simulink library "CoCoSTLib"  (R2021a)
settings: Solver=ode45  StartTime=0.0  StopTime=10.0  RelTol=1e-3  EnableMultiTasking=on
values from neighbouring files (symbols this model uses):
  beta = 0.01    [var.mat]
  c = 2    [var.mat]
  m = 4    [var.mat]
  mu = 0.8    [var.mat]
  omega = 1    [var.mat]
  r = 5    [var.mat]
  s = 1.5    [var.mat]
  steadyVal = 10    [var.mat]
  zeta = 0.5    [var.mat]
undefined symbols (not defined in the file or in its folder): a, d, msgbox, T_End, T_Start, tau
libraries: $bdroot x49, simulink x4
(part 1 of 2)
settings Model: Creator=balsi  LastModifiedBy=xiayu
settings SolverCC: AlgebraicLoopSolver=TrustRegion
settings DataIOCC: LimitDataPoints=on  SaveFormat=Array  ReturnWorkspaceOutputs=off
settings OptimizationCC: LifeSpan=inf
settings DebuggingCC: SFUnexpectedBacktrackingDiag=warning  SFNoUnconditionalDefaultTransitionDiag=warning  SFExecutionAtInitializationDiag=none  SFMachineParentedDataDiag=warning  ArithmeticOperatorsInVariantConditions=warning
settings HardwareCC: ProdBitPerPointer=32  ProdBitPerSizeT=32  ProdBitPerPtrDiffT=32  ProdLargestAtomicFloat=None  ProdIntDivRoundTo=Undefined  ProdEndianess=Unspecified  ProdWordSize=32  ProdHWDeviceType=32-bit Generic
settings ModelReferenceCC: PropagateSignalLabelsOutOfModel=off
settings SFSimCC: SimUseLocalCustomCode=off  CustomCodeUndefinedFunction=UseInterfaceOnly
settings RTWCC: RTWUseLocalCustomCode=off
settings CodeAppCC: StateflowObjectComments=on
settings GRTTargetCC: TargetLangStandard=C89/C90 (ANSI)
settings ConfigComp: CovMetricSettings=dw  CovSaveCumulativeToWorkspaceVar=on  CovSaveSingleToWorkspaceVar=on  CovExternalEMLEnable=off

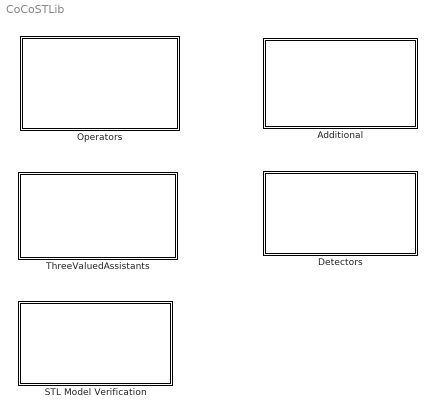
== system CoCoSTLib ==
  Additional : Subsystem
      mask Display: disp('Some Utiles')
  Detectors : Subsystem
      mask Display: disp("Detectors")
  Operators : Subsystem
      mask Display: disp("STL Operators")
  STL Model Verification : Subsystem
      mask Display: disp("STL Model Verification")
  ThreeValuedAssistants : Subsystem
      mask Display: disp("Utiles for 3V Logic")

== system CoCoSTLib/Additional ==
  note: Time Windows
  note: Latches
  note: AndSTL
  note: Delay
  AndStl_LF : Subsystem
  AndStl_LT : Subsystem
  Delay : Subsystem
  DelayedTimeWindow : Subsystem
  Latch_LF : Subsystem
  Latch_LT : Subsystem
  TimeWindow : Subsystem

== system CoCoSTLib/Detectors ==
  note: Detectors of Unaccepted signal behaviors
      |
      | - Components are in LT framework.
      | - The detectors/monitors definitions are in S T - Lib : A library for specifying and classifying model behaviors
  Overshoot : Subsystem  mask{c=c, r=r}
      mask prompts: c "Overshoot magnitude"; r "Step parameter"
      mask TypeOptions c: c/Value
      mask TypeOptions r:
      | r
      | /Value
  Ring_once : Subsystem  mask{a=a, d=2*d}
      mask prompts: a "amplitude of the ring"; d "maximum width of the ring"
      mask TypeOptions a: a/Value
      mask TypeOptions d: d/Value
  RiseTime : Subsystem  mask{r=r, zeta=zeta, value=mu * steadyVal}
      mask prompts: r "Step parameter"; zeta "Rise time"; value "Target value to reach"
      mask TypeOptions r: r/Value
      mask TypeOptions zeta: zeta/Value
      mask TypeOptions value: target value/Value
  SettlingTime : Subsystem  mask{r=r, s=s, beta=beta}
      mask prompts: r "Step parameter"; s "Settling time"; beta "Fraction of steady state value"
      mask TypeOptions r:
      | r
      | /Value
      mask TypeOptions s: s/Value
      mask TypeOptions beta: beta/Gain
  Spike : Subsystem  mask{m=m, omega=omega}
      mask prompts: m "amplitude of spike"; omega "maximum width of spike"
      mask TypeOptions m: m/Value
      mask TypeOptions omega: omega/Value
  Timed Relationship : Subsystem  mask{tau=tau}
      mask prompts: tau "Relation time"
      mask TypeOptions tau: tau/Value

== system CoCoSTLib/Operators ==
  Operators_3V : Subsystem
      mask Display: disp("Operators Three-valued Logic")
  Operators_LF : Subsystem
      mask Display: disp('Operators True Logic')
  Operators_LT : Subsystem
      mask Display: disp('Operators False Logic')

== system CoCoSTLib/STL Model Verification ==
  note: 3V assertion
  note: 3V indicator/bulb
  3V Assertion : Subsystem  mask(Assertion in Three-valued Logic){Enabled=on, AssertionFailFcn=, StopWhenAssertionFail=on}
      mask prompts: Enabled "Simulink:blkprm_prompts:AssertionEnabled"; AssertionFailFcn "Simulink:blkprm_prompts:AssertionCallback"; StopWhenAssertionFail "Simulink:blkprm_prompts:AssertionStopRequest"
      mask help:
      | The Assertion block checks whether any of the elements of the input signal are of FALSE value in Three-Valued Logic,  namely [0, 0]. If all elements are nonzero, the block does nothing. If any element is zero, the block halts the simulation, by default, and displays an error message.
      |
      | NOTE: This block is used when 3V encoding is [0, 0], [0, 1], [1, 0], [1, 1]. When 3V encoding is -1, 0, 1, use Simulink / Model Verification / Assertion.
      mask TypeOptions Enabled: Assertion/Enabled
      mask TypeOptions AssertionFailFcn: Assertion/AssertionFailFcn
      mask TypeOptions StopWhenAssertionFail: Assertion/StopWhenAssertionFail
      mask DialogControl Enabled Prompt: Enable assertion
      mask DialogControl AssertionFailFcn Prompt: Simulation callback when assertion fails:
      mask DialogControl StopWhenAssertionFail Prompt: Stop simulation when assertion fails
  3V Lamp : LampBlock
  report : Subsystem  StopFcn=msgbox('msg here', 'report');

== system CoCoSTLib/ThreeValuedAssistants ==
  note: Encoding of 3V Logic in -1, 0, 1
  note: 3V interpreter
  note: 3V assignments
  note: 3V logic operators
  AND_3V : Subsystem
  Assignment_arr : Subsystem  Commented=on
  False_3V : Subsystem
      mask Display: disp("F_3V")
  "Interpreter " : Subsystem
  NOT_3V : Subsystem
  OR_3V : Subsystem
  True_3V : Subsystem
      mask Display: disp("T_3V")
  Unknown_3V : Subsystem
      mask Display: disp("U_3V")

== system CoCoSTLib/Additional/AndStl_LF ==
  note: This block gives the time when IN has an decrease, i.e, the value of the delay
  IN : Inport
  Clock : Clock
  Constant : Constant  Value=65535  VectorParams1D=off
  Constant1 : Constant
  DetectDecrease : Subsystem
  Memory : Memory
  Memory1 : Memory
  Switch : Switch  Criteria=u2 > Threshold
  Switch1 : Switch  Criteria=u2 > Threshold
  Switch2 : Switch  Criteria=u2 > Threshold
  OUT : Outport
  wires:
  Memory1/1 -> Switch1/2, Switch2/3
  Switch/1 -> Memory/1
  Memory/1 -> Switch1/1, Switch/3
  Switch1/1 -> OUT/1
  Switch2/1 -> Memory1/1
  Clock/1 -> Switch/1
  DetectDecrease/1(Y) -> Switch/2, Switch2/2
  Constant/1 -> Switch1/3
  IN/1 -> DetectDecrease/1(U)
  Constant1/1 -> Switch2/1

== system CoCoSTLib/Additional/AndStl_LT ==
  note: This block gives the time when IN has an increase, i.e, the value of the delay
  IN : Inport
  Clock : Clock
  Constant : Constant  Value=65535
  Constant1 : Constant
  DetectIncrease : Subsystem
  Memory : Memory
  Memory1 : Memory
  Switch : Switch  Criteria=u2 > Threshold
  Switch1 : Switch  Criteria=u2 > Threshold
  Switch2 : Switch  Criteria=u2 > Threshold
  OUT : Outport
  wires:
  Clock/1 -> Switch/1
  Constant1/1 -> Switch2/1
  Memory1/1 -> Switch1/2, Switch2/3
  Switch/1 -> Memory/1
  Switch1/1 -> OUT/1
  Switch2/1 -> Memory1/1
  DetectIncrease/1(Y) -> Switch/2, Switch2/2
  IN/1 -> DetectIncrease/1(U)
  Memory/1 -> Switch1/1, Switch/3
  Constant/1 -> Switch1/3

== system CoCoSTLib/Additional/Delay ==
  T_Start : Inport
  T_End : Inport  Port=2
  Delay : Inport  Port=3
  Clock : Clock
  Compare To Constant : simulink/Logic and Bit Operations/Compare To Constant  relop=>=  const=0  OutDataTypeStr=boolean
  Constant : Constant  Value=65535
  Subtract : Sum
  Subtract1 : Sum
  Subtract2 : Sum  Inputs=-+
  Switch1 : Switch  Criteria=u2 > Threshold
  T_Start_delayed : Outport
  T_End_delayed : Outport  Port=2
  wires:
  Clock/1 -> Subtract2/2
  Constant/1 -> Switch1/3
  Switch1/1 -> Subtract/1, Subtract1/2
  Delay/1 -> Switch1/1, Subtract2/1
  T_End/1 -> Subtract1/1
  T_Start/1 -> Subtract/2
  Subtract1/1 -> T_End_delayed/1
  Subtract/1 -> T_Start_delayed/1
  Subtract2/1 -> Compare To Constant/1
  Compare To Constant/1 -> Switch1/2

== system CoCoSTLib/Additional/DelayedTimeWindow ==
  T_Start : Inport
  T_End : Inport  Port=2
  DELAY : Inport  Port=3
  AND1 : Logic  AllPortsSameDT=off  OutDataTypeStr=boolean
  CLOCK : Clock
  DELAY_SUB : Sum  Inputs=+-
  REL1 : RelationalOperator  Operator=<=  OutDataTypeStr=boolean  RndMeth=Simplest
  REL2 : RelationalOperator  Operator=<=  OutDataTypeStr=boolean  RndMeth=Simplest
  OUT : Outport
  wires:
  REL1/1 -> AND1/1
  CLOCK/1 -> DELAY_SUB/1
  REL2/1 -> AND1/2
  T_Start/1 -> REL1/1
  DELAY_SUB/1 -> REL1/2, REL2/1
  AND1/1 -> OUT/1
  DELAY/1 -> DELAY_SUB/2
  T_End/1 -> REL2/2

== system CoCoSTLib/Additional/Latch_LF ==
  In : Inport
  Memory_ini1 : Memory  InitialCondition=1
  OR : Logic  AllPortsSameDT=off  OutDataTypeStr=boolean
  Out : Outport
  wires:
  In/1 -> OR/1
  Memory_ini1/1 -> OR/2
  OR/1 -> Out/1, Memory_ini1/1

== system CoCoSTLib/Additional/Latch_LT ==
  In : Inport
  "Memory_ini0 " : Memory
  OR : Logic  Operator=OR  AllPortsSameDT=off  OutDataTypeStr=boolean
  Out : Outport
  wires:
  In/1 -> OR/1
  "Memory_ini0 "/1 -> OR/2
  OR/1 -> Out/1, "Memory_ini0 "/1

== system CoCoSTLib/Additional/TimeWindow ==
  T_Start : Inport
  T_End : Inport  Port=2
  AND : Logic  AllPortsSameDT=off  OutDataTypeStr=boolean
  CLOCK : Clock
  REL1 : RelationalOperator  Operator=<=  OutDataTypeStr=boolean  RndMeth=Simplest
  REL2 : RelationalOperator  Operator=<=  OutDataTypeStr=boolean  RndMeth=Simplest
  OUT : Outport
  wires:
  CLOCK/1 -> REL1/2, REL2/1
  T_End/1 -> REL2/2
  REL1/1 -> AND/1
  REL2/1 -> AND/2
  AND/1 -> OUT/1
  T_Start/1 -> REL1/1

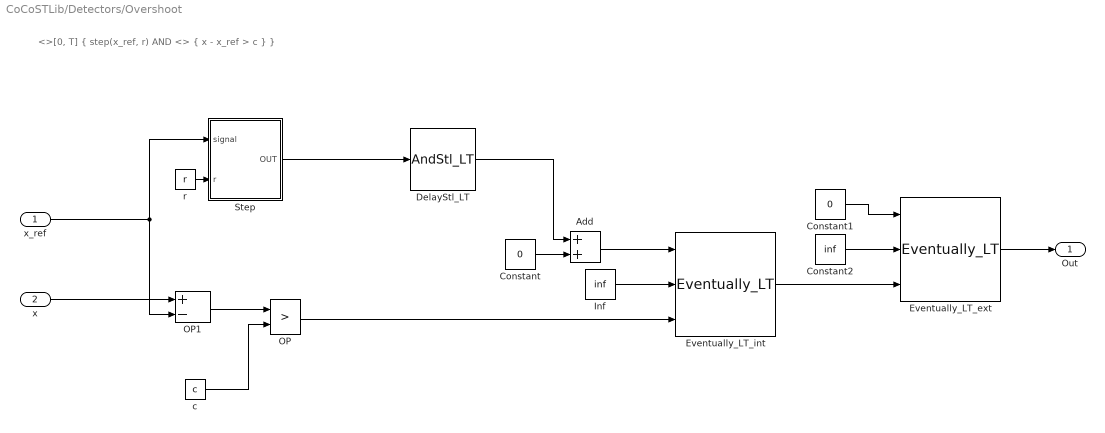
== system CoCoSTLib/Detectors/Overshoot ==
  note: <>[0, T] { step(x_ref, r) AND <> { x - x_ref > c } }
  x_ref : Inport
  x : Inport  Port=2
  Add : Sum
  Constant : Constant  Value=0
  Constant1 : Constant  Value=0
  Constant2 : Constant  Value=inf
  DelayStl_LT : $bdroot/Additional/AndStl_LT  SystemSampleTime=-1  VariantActivationTime=update diagram  Latency=0  AutoFrameSizeCalculation=off
  Eventually_LT_ext : $bdroot/Operators/Operators_LT/Eventually_LT   SystemSampleTime=-1  VariantActivationTime=update diagram  Latency=0  AutoFrameSizeCalculation=off
  "Eventually_LT_int " : $bdroot/Operators/Operators_LT/Eventually_LT   SystemSampleTime=-1  VariantActivationTime=update diagram  Latency=0  AutoFrameSizeCalculation=off
  Inf : Constant  Value=inf  OutDataTypeStr=Inherit: Inherit via back propagation
  OP : RelationalOperator  Operator=>  OutDataTypeStr=boolean  RndMeth=Simplest
  OP1 : Sum  Inputs=+-
  "Step " : Subsystem
  c : Constant  Value=c
  "r " : Constant  Value=r
  Out : Outport
  wires:
  x_ref/1 -> "Step "/1(signal), OP1/2
  DelayStl_LT/1 -> Add/1
  x/1 -> OP1/1
  Add/1 -> "Eventually_LT_int "/1
  "Step "/1(OUT) -> DelayStl_LT/1
  Eventually_LT_ext/1 -> Out/1
  "r "/1 -> "Step "/2(r)
  Constant/1 -> Add/2
  Inf/1 -> "Eventually_LT_int "/2
  c/1 -> OP/2
  Constant1/1 -> Eventually_LT_ext/1
  Constant2/1 -> Eventually_LT_ext/2
  "Eventually_LT_int "/1 -> Eventually_LT_ext/3
  OP1/1 -> OP/1
  OP/1 -> "Eventually_LT_int "/3

== system CoCoSTLib/Detectors/Ring_once ==
  note: <>[0, T] (rise and <>_[0, 2d] fall)
  signal : Inport
  "AndSTL_LT " : $bdroot/Additional/AndStl_LT  SystemSampleTime=-1  VariantActivationTime=update diagram  Latency=0  AutoFrameSizeCalculation=off
  Constant : Constant  Value=0
  "Eventually_LT " : $bdroot/Operators/Operators_LT/Eventually_LT   SystemSampleTime=-1  VariantActivationTime=update diagram  Latency=0  AutoFrameSizeCalculation=off
  Fall : Subsystem
  Rise : Subsystem
  Subtract : Sum
  Subtract1 : Sum
  a : Constant  Value=a
  d : Constant  Value=d
  "out " : Outport
  wires:
  "AndSTL_LT "/1 -> Subtract/1, Subtract1/2
  Constant/1 -> Subtract/2
  d/1 -> Subtract1/1
  Subtract/1 -> "Eventually_LT "/1
  Subtract1/1 -> "Eventually_LT "/2
  Rise/1(OUT) -> "AndSTL_LT "/1
  "Eventually_LT "/1 -> "out "/1
  signal/1 -> Fall/1(signal), Rise/1(signal)  "signal"
  Fall/1(OUT) -> "Eventually_LT "/3
  a/1 -> Rise/2("a "), Fall/2(a)

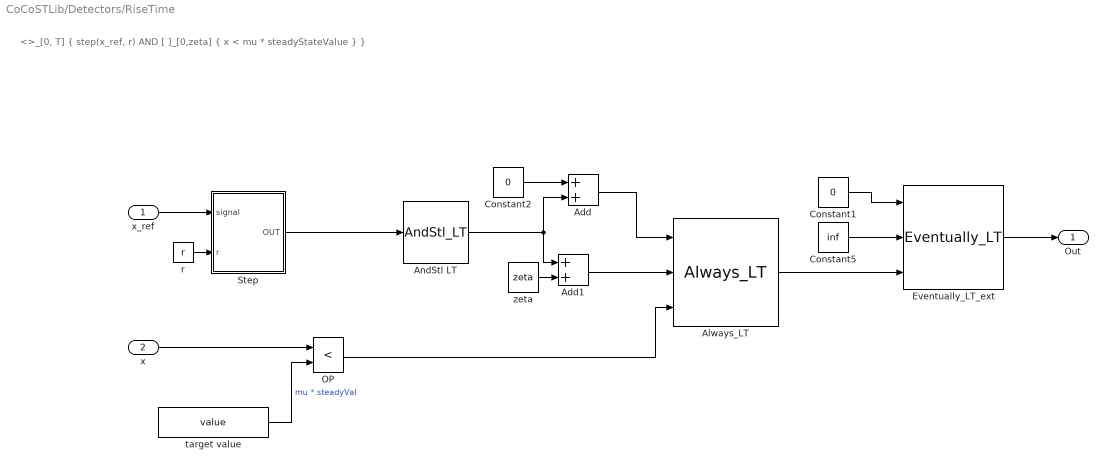
== system CoCoSTLib/Detectors/RiseTime ==
  note: <>_[0, T] { step(x_ref, r) AND [ ]_[0,zeta] { x < mu * steadyStateValue } }
  "x_ref " : Inport
  x : Inport  Port=2
  Add : Sum
  Add1 : Sum
  "Always_LT " : $bdroot/Operators/Operators_LT/Always_LT   SystemSampleTime=-1  VariantActivationTime=update diagram  Latency=0  AutoFrameSizeCalculation=off
  AndStl LT : $bdroot/Additional/AndStl_LT  SystemSampleTime=-1  VariantActivationTime=update diagram  Latency=0  AutoFrameSizeCalculation=off
  Constant1 : Constant  Value=0
  Constant2 : Constant  Value=0
  Constant5 : Constant  Value=inf
  Eventually_LT_ext : $bdroot/Operators/Operators_LT/Eventually_LT   SystemSampleTime=-1  VariantActivationTime=update diagram  Latency=0  AutoFrameSizeCalculation=off
  OP : RelationalOperator  Operator=<  OutDataTypeStr=boolean  RndMeth=Simplest
  "Step " : Subsystem
  r : Constant  Value=r
  target value : Constant  Value=value
  zeta : Constant  Value=zeta
  Out : Outport
  wires:
  r/1 -> "Step "/2(r)
  target value/1 -> OP/2  "mu * steadyVal"
  Eventually_LT_ext/1 -> Out/1
  "x_ref "/1 -> "Step "/1(signal)
  x/1 -> OP/1
  OP/1 -> "Always_LT "/3
  Constant5/1 -> Eventually_LT_ext/2
  "Always_LT "/1 -> Eventually_LT_ext/3
  Constant1/1 -> Eventually_LT_ext/1
  "Step "/1(OUT) -> AndStl LT/1
  Constant2/1 -> Add/1
  Add/1 -> "Always_LT "/1
  zeta/1 -> Add1/2
  Add1/1 -> "Always_LT "/2
  AndStl LT/1 -> Add/2, Add1/1

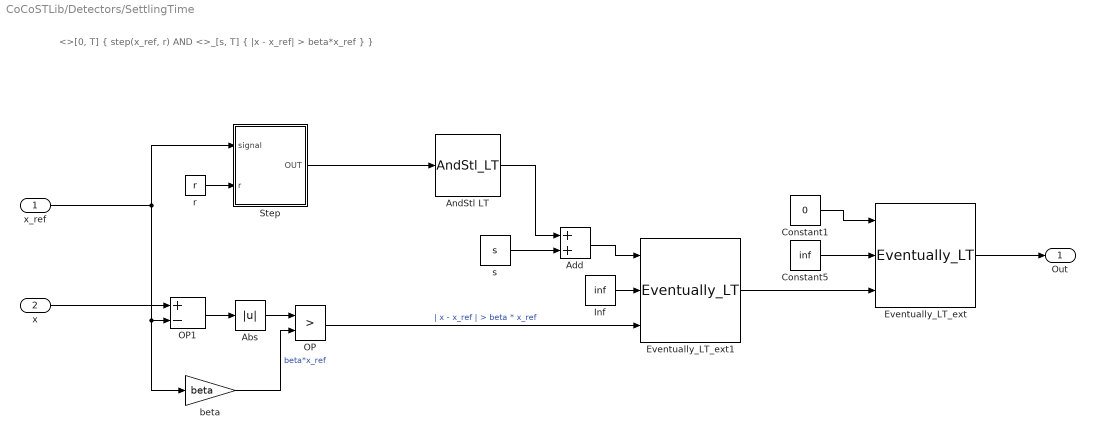
== system CoCoSTLib/Detectors/SettlingTime ==
  note: <>[0, T] { step(x_ref, r) AND <>_[s, T] { |x - x_ref| > beta*x_ref } }
  x_ref : Inport
  x : Inport  Port=2
  Abs : Abs
  Add : Sum
  AndStl LT : $bdroot/Additional/AndStl_LT  SystemSampleTime=-1  VariantActivationTime=update diagram  Latency=0  AutoFrameSizeCalculation=off
  Constant1 : Constant  Value=0
  Constant5 : Constant  Value=inf
  Eventually_LT_ext : $bdroot/Operators/Operators_LT/Eventually_LT   SystemSampleTime=-1  VariantActivationTime=update diagram  Latency=0  AutoFrameSizeCalculation=off
  Eventually_LT_ext1 : $bdroot/Operators/Operators_LT/Eventually_LT   SystemSampleTime=-1  VariantActivationTime=update diagram  Latency=0  AutoFrameSizeCalculation=off
  Inf : Constant  Value=inf  OutDataTypeStr=Inherit: Inherit via back propagation
  OP : RelationalOperator  Operator=>  OutDataTypeStr=boolean  RndMeth=Simplest
  OP1 : Sum  Inputs=+-
  "Step " : Subsystem
  beta : Gain  Gain=beta
  "r " : Constant  Value=r
  s : Constant  Value=s
  Out : Outport
  wires:
  beta/1 -> OP/2  "beta*x_ref"
  Abs/1 -> OP/1
  "r "/1 -> "Step "/2(r)
  OP/1 -> Eventually_LT_ext1/3  "| x - x_ref | > beta * x_ref"
  x/1 -> OP1/1
  Eventually_LT_ext/1 -> Out/1
  x_ref/1 -> beta/1, OP1/2, "Step "/1(signal)
  OP1/1 -> Abs/1
  Constant1/1 -> Eventually_LT_ext/1
  Constant5/1 -> Eventually_LT_ext/2
  Eventually_LT_ext1/1 -> Eventually_LT_ext/3
  "Step "/1(OUT) -> AndStl LT/1
  Inf/1 -> Eventually_LT_ext1/2
  Add/1 -> Eventually_LT_ext1/1
  AndStl LT/1 -> Add/1
  s/1 -> Add/2

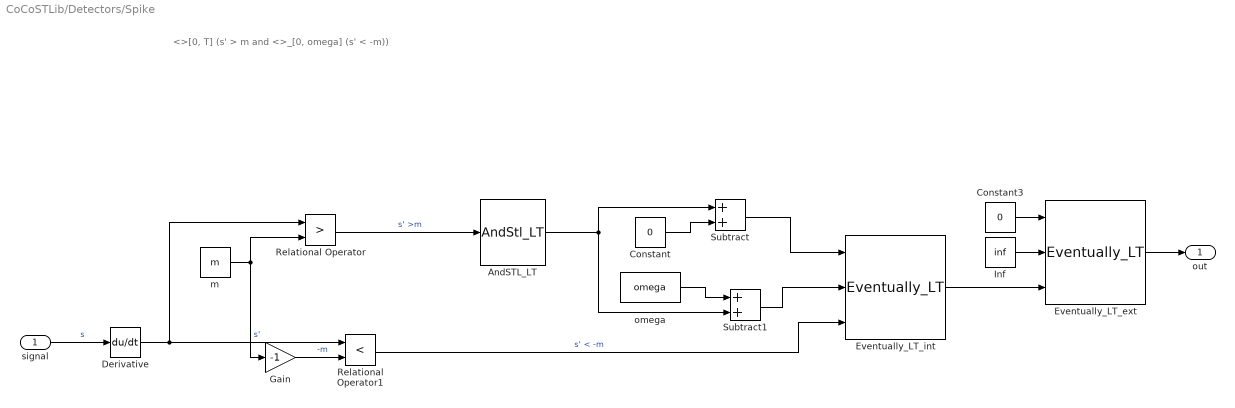
== system CoCoSTLib/Detectors/Spike ==
  note: <>[0, T] (s' > m and <>_[0, omega] (s' < -m))
  signal : Inport
  "AndSTL_LT " : $bdroot/Additional/AndStl_LT  SystemSampleTime=-1  VariantActivationTime=update diagram  Latency=0  AutoFrameSizeCalculation=off
  Constant : Constant  Value=0
  Constant3 : Constant  Value=0
  Derivative : Derivative
  Eventually_LT_ext : $bdroot/Operators/Operators_LT/Eventually_LT   SystemSampleTime=-1  VariantActivationTime=update diagram  Latency=0  AutoFrameSizeCalculation=off
  "Eventually_LT_int " : $bdroot/Operators/Operators_LT/Eventually_LT   SystemSampleTime=-1  VariantActivationTime=update diagram  Latency=0  AutoFrameSizeCalculation=off
  Gain : Gain  Gain=-1
  Inf : Constant  Value=inf  OutDataTypeStr=Inherit: Inherit via back propagation
  Relational Operator : RelationalOperator  Operator=>  OutDataTypeStr=boolean  RndMeth=Simplest
  Relational Operator1 : RelationalOperator  Operator=<  OutDataTypeStr=boolean  RndMeth=Simplest
  Subtract : Sum
  Subtract1 : Sum
  m : Constant  Value=m
  omega : Constant  Value=omega
  "out " : Outport
  wires:
  signal/1 -> Derivative/1  "s"
  Eventually_LT_ext/1 -> "out "/1
  Constant3/1 -> Eventually_LT_ext/1
  "Eventually_LT_int "/1 -> Eventually_LT_ext/3
  Gain/1 -> Relational Operator1/2  "-m"
  Derivative/1 -> Relational Operator1/1, Relational Operator/1  "s'"
  m/1 -> Relational Operator/2, Gain/1
  Relational Operator1/1 -> "Eventually_LT_int "/3  "s' < -m"
  "AndSTL_LT "/1 -> Subtract/1, Subtract1/2
  Constant/1 -> Subtract/2
  omega/1 -> Subtract1/1
  Subtract/1 -> "Eventually_LT_int "/1
  Subtract1/1 -> "Eventually_LT_int "/2
  Inf/1 -> Eventually_LT_ext/2
  Relational Operator/1 -> "AndSTL_LT "/1  "s' >m"

== system CoCoSTLib/Detectors/Timed Relationship ==
  note: <>_[0, T]{ p1 AND [ ]_[0,tau] not p2 }
  "p1 " : Inport
  p2 : Inport  Port=2
  Add : Sum
  Add1 : Sum
  "Always_LT " : $bdroot/Operators/Operators_LT/Always_LT   SystemSampleTime=-1  VariantActivationTime=update diagram  Latency=0  AutoFrameSizeCalculation=off
  AndStl LT : $bdroot/Additional/AndStl_LT  SystemSampleTime=-1  VariantActivationTime=update diagram  Latency=0  AutoFrameSizeCalculation=off
  Constant1 : Constant  Value=0
  Constant2 : Constant  Value=0
  Constant5 : Constant  Value=inf
  Eventually_LT_ext : $bdroot/Operators/Operators_LT/Eventually_LT   SystemSampleTime=-1  VariantActivationTime=update diagram  Latency=0  AutoFrameSizeCalculation=off
  NOT : Logic  Operator=NOT  IconShape=distinctive  AllPortsSameDT=off  OutDataTypeStr=boolean
  tau : Constant  Value=tau
  Out : Outport
  wires:
  Eventually_LT_ext/1 -> Out/1
  Constant5/1 -> Eventually_LT_ext/2
  "Always_LT "/1 -> Eventually_LT_ext/3
  Constant1/1 -> Eventually_LT_ext/1
  "p1 "/1 -> AndStl LT/1
  Constant2/1 -> Add/1
  Add/1 -> "Always_LT "/1
  tau/1 -> Add1/2
  Add1/1 -> "Always_LT "/2
  AndStl LT/1 -> Add/2, Add1/1
  p2/1 -> NOT/1
  NOT/1 -> "Always_LT "/3

== system CoCoSTLib/Operators/Operators_3V ==
  Always_3V : Subsystem
  Eventually_3V : Subsystem
  Until_3V : Subsystem

== system CoCoSTLib/Operators/Operators_LF ==
  AlwaysLF mfunction : MATLAB Function  Commented=on  TreatAsAtomicUnit=on
  Always_LF : Subsystem
  Always_LF_delay : Subsystem
  Always_LF_param : Subsystem  mask{T_Start=T_Start, T_End=T_End}
      mask prompts: T_Start "T_Start Value"; T_End "T_End Value"
      mask TypeOptions T_Start: T_Start/Value
      mask TypeOptions T_End: T_End/Value
  Eventually_LF : Subsystem
  Eventually_LF_param : Subsystem  mask{T_Start=T_Start, T_End=T_End}
      mask prompts: T_Start "T_Start Value"; T_End "T_End Value"
      mask TypeOptions T_Start: T_Start/Value
      mask TypeOptions T_End: T_End/Value
  Eventually_LFbis : Subsystem  Commented=on
  Until_LF : Subsystem
  Until_LF_param : Subsystem  mask{T_Start=T_Start, T_End=T_End}
      mask TypeOptions T_Start: T_Start/Value
      mask TypeOptions T_End: T_End/Value

== system CoCoSTLib/Operators/Operators_LT ==
  "Always_LT " : Subsystem
  Always_LT_timewindow : Subsystem
  Always_LTbis : Subsystem  Commented=on
  "Eventually_LT " : Subsystem
  Eventually_LT bis : Subsystem  Commented=on
  Eventually_LT_timewindow : Subsystem
  Until_LT : Subsystem

== system CoCoSTLib/STL Model Verification/3V Assertion ==
  In : Inport
  AND : Logic  Operator=OR  IconShape=distinctive  AllPortsSameDT=off  OutDataTypeStr=boolean
  Assertion : Assertion
  Compare To Constant : simulink/Logic and Bit Operations/Compare To Constant  relop=~=  const=0  OutDataTypeStr=boolean
  Compare To Constant1 : simulink/Logic and Bit Operations/Compare To Constant  relop=~=  const=0  OutDataTypeStr=boolean
  Demux : Demux  Outputs=2
  wires:
  Demux/1 -> Compare To Constant/1
  AND/1 -> Assertion/1
  Compare To Constant1/1 -> AND/2
  Compare To Constant/1 -> AND/1
  In/1 -> Demux/1
  Demux/2 -> Compare To Constant1/1

== system CoCoSTLib/STL Model Verification/report ==
  simout : Inport
  Terminator : Terminator
  wires:
  simout/1 -> Terminator/1

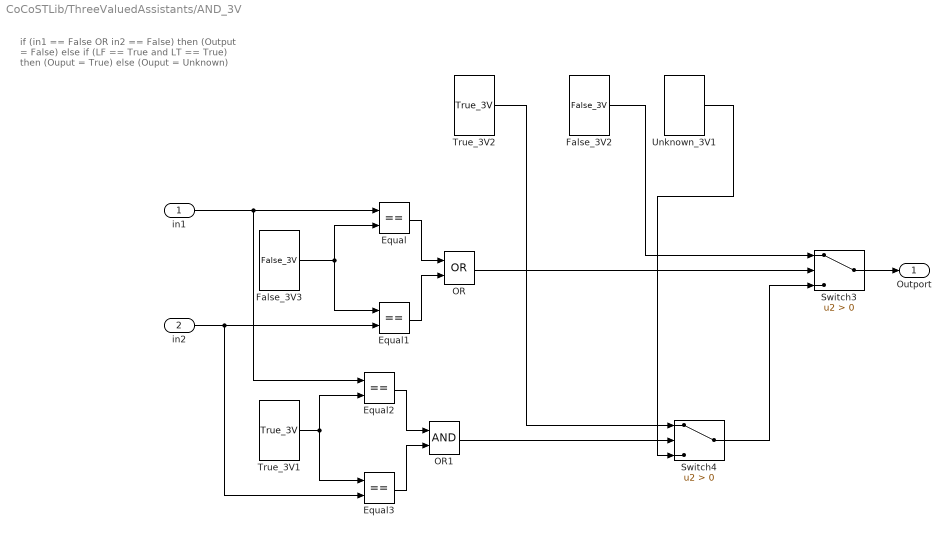
== system CoCoSTLib/ThreeValuedAssistants/AND_3V ==
  note: if (in1 == False OR in2 == False)
      | then (Output = False)
      | else if (LF == True and LT == True)
      | then (Ouput = True)
      | else (Ouput = Unknown)
  "in1 " : Inport
  in2 : Inport  Port=2
  Equal{,1..3} (4 alike) : RelationalOperator  Operator===  OutDataTypeStr=boolean  RndMeth=Simplest
  False_3V2 : $bdroot/ThreeValuedAssistants/False_3V  SystemSampleTime=-1  VariantActivationTime=update diagram  Latency=0  AutoFrameSizeCalculation=off
  False_3V3 : $bdroot/ThreeValuedAssistants/False_3V  SystemSampleTime=-1  VariantActivationTime=update diagram  Latency=0  AutoFrameSizeCalculation=off
  OR : Logic  Operator=OR  AllPortsSameDT=off  OutDataTypeStr=boolean
  OR1 : Logic  AllPortsSameDT=off  OutDataTypeStr=boolean
  Switch3 : Switch  Criteria=u2 > Threshold
  Switch4 : Switch  Criteria=u2 > Threshold
  True_3V1 : $bdroot/ThreeValuedAssistants/True_3V  SystemSampleTime=-1  VariantActivationTime=update diagram  Latency=0  AutoFrameSizeCalculation=off
  True_3V2 : $bdroot/ThreeValuedAssistants/True_3V  SystemSampleTime=-1  VariantActivationTime=update diagram  Latency=0  AutoFrameSizeCalculation=off
  Unknown_3V1 : $bdroot/ThreeValuedAssistants/Unknown_3V  SystemSampleTime=-1  VariantActivationTime=update diagram  Latency=0  AutoFrameSizeCalculation=off
  Outport : Outport
  wires:
  False_3V3/1 -> Equal/2, Equal1/1
  Equal/1 -> OR/1
  Equal1/1 -> OR/2
  OR/1 -> Switch3/2
  Switch3/1 -> Outport/1
  Equal2/1 -> OR1/1
  Equal3/1 -> OR1/2
  OR1/1 -> Switch4/2
  "in1 "/1 -> Equal2/1, Equal/1
  True_3V1/1 -> Equal2/2, Equal3/1
  in2/1 -> Equal1/2, Equal3/2
  True_3V2/1 -> Switch4/1
  Switch4/1 -> Switch3/3
  False_3V2/1 -> Switch3/1
  Unknown_3V1/1 -> Switch4/3

== system CoCoSTLib/ThreeValuedAssistants/Assignment_arr ==
  note: In order to save memory, values can be encoded in two digits.
      | For example:
      | 	True: [1, 1]
      |        False: [ 0, 0]
      |        Unknown: [1, 0]
  Cast To Boolean : DataTypeConversion  Commented=on  OutDataTypeStr=boolean
  Cast To Boolean1 : DataTypeConversion  Commented=on  OutDataTypeStr=boolean
  Cast To Boolean2 : DataTypeConversion  Commented=on  OutDataTypeStr=boolean
  Constant : Constant  Commented=on
  Constant1 : Constant  Commented=on  Value=0
  Constant2 : Constant  Commented=on
  Constant3 : Constant  Commented=on  Value=0
  Constant4 : Constant  Commented=on
  Constant5 : Constant  Commented=on  Value=0
  False_3V1 : Subsystem
      mask Display: disp("F_3V")
  Mux : Mux  Commented=on  Inputs=2
  Mux1 : Mux  Commented=on  Inputs=2
  Mux2 : Mux  Commented=on  Inputs=2
  Ture_3V : Subsystem
      mask Display: disp("T_3V")
  Unknown_3V1 : Subsystem
      mask Display: disp("U_3V")
  wires:
  Constant5/1 -> Mux2/2
  Mux1/1 -> Cast To Boolean1/1
  Constant3/1 -> Mux1/2
  Cast To Boolean1/1 -> ?
  Unknown_3V1/1(Outport) -> ?
  Cast To Boolean/1 -> ?
  False_3V1/1(Outport) -> ?
  Mux2/1 -> Cast To Boolean2/1
  Ture_3V/1(Outport) -> ?
  Constant2/1 -> Mux/2
  Cast To Boolean2/1 -> ?
  Mux/1 -> Cast To Boolean/1
  Constant/1 -> Mux/1
  Constant4/1 -> Mux2/1
  Constant1/1 -> Mux1/1

== system CoCoSTLib/ThreeValuedAssistants/False_3V ==
  Constant1 : Constant  Value=0
  Out1 : Outport
  wires:
  Constant1/1 -> Out1/1

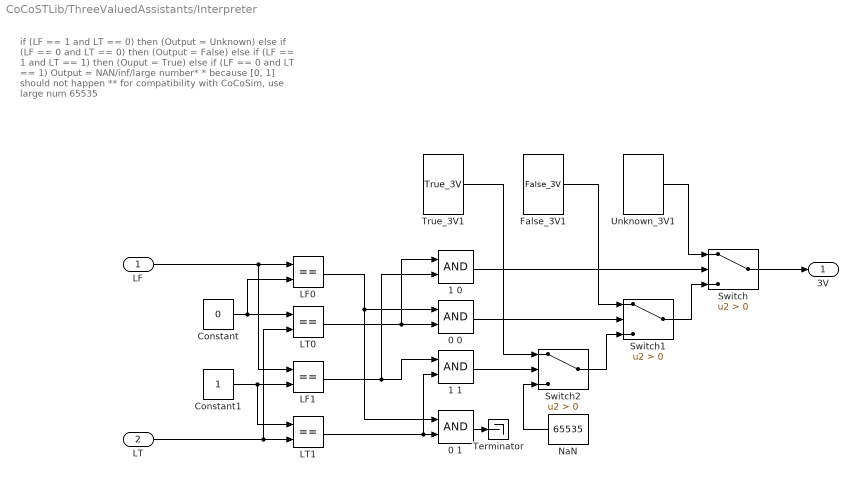
== system CoCoSTLib/ThreeValuedAssistants/Interpreter  ==
  note: if (LF == 1 and LT == 0)
      | then (Output = Unknown)
      | else if (LF == 0 and LT == 0)
      | then (Output = False)
      | else if (LF == 1 and LT == 1)
      | then (Ouput = True)
      | else if (LF == 0 and LT == 1)
      | Output = NAN/inf/large number*
      |
      | * because [0, 1] should not happen
      | ** for compatibility with CoCoSim, use large num 65535
  LF : Inport
  LT : Inport  Port=2
  0 0 : Logic  AllPortsSameDT=off  OutDataTypeStr=boolean
  0 1 : Logic  AllPortsSameDT=off  OutDataTypeStr=boolean
  1 0 : Logic  AllPortsSameDT=off  OutDataTypeStr=boolean
  1 1 : Logic  AllPortsSameDT=off  OutDataTypeStr=boolean
  Constant : Constant  Value=0
  Constant1 : Constant
  False_3V1 : $bdroot/ThreeValuedAssistants/False_3V  SystemSampleTime=-1  VariantActivationTime=update diagram  Latency=0  AutoFrameSizeCalculation=off
  LF0 : RelationalOperator  Operator===  OutDataTypeStr=boolean  RndMeth=Simplest
  LF1 : RelationalOperator  Operator===  OutDataTypeStr=boolean  RndMeth=Simplest
  "LT0 " : RelationalOperator  Operator===  OutDataTypeStr=boolean  RndMeth=Simplest
  "LT1 " : RelationalOperator  Operator===  OutDataTypeStr=boolean  RndMeth=Simplest
  NaN : Constant  Value=65535  OutDataTypeStr=Inherit: Inherit via back propagation
  Switch : Switch  Criteria=u2 > Threshold
  Switch1 : Switch  Criteria=u2 > Threshold
  Switch2 : Switch  Criteria=u2 > Threshold
  Terminator : Terminator
  True_3V1 : $bdroot/ThreeValuedAssistants/True_3V  SystemSampleTime=-1  VariantActivationTime=update diagram  Latency=0  AutoFrameSizeCalculation=off
  Unknown_3V1 : $bdroot/ThreeValuedAssistants/Unknown_3V  SystemSampleTime=-1  VariantActivationTime=update diagram  Latency=0  AutoFrameSizeCalculation=off
  3V : Outport
  wires:
  Constant/1 -> "LT0 "/1, LF0/2
  1 0/1 -> Switch/2
  Switch/1 -> 3V/1
  Constant1/1 -> LF1/2, "LT1 "/1
  LF1/1 -> 1 1/1, 1 0/2
  0 0/1 -> Switch1/2
  Switch1/1 -> Switch/3
  "LT0 "/1 -> 0 0/2, 1 0/1
  LF0/1 -> 0 1/1, 0 0/1
  "LT1 "/1 -> 1 1/2, 0 1/2
  1 1/1 -> Switch2/2
  Switch2/1 -> Switch1/3
  0 1/1 -> Terminator/1
  NaN/1 -> Switch2/3
  Unknown_3V1/1 -> Switch/1
  True_3V1/1 -> Switch2/1
  False_3V1/1 -> Switch1/1
  LF/1 -> LF1/1, LF0/1
  LT/1 -> "LT0 "/2, "LT1 "/2

== system CoCoSTLib/ThreeValuedAssistants/NOT_3V ==
  note: if (in == True)
      | then (Output = False)
      | else if (in == False)
      | then (Ouput = True)
      | else (Ouput = Unknown)
  "Input " : Inport
  Equal : RelationalOperator  Operator===  OutDataTypeStr=boolean  RndMeth=Simplest
  Equal2 : RelationalOperator  Operator===  OutDataTypeStr=boolean  RndMeth=Simplest
  False_3V1 : $bdroot/ThreeValuedAssistants/False_3V  SystemSampleTime=-1  VariantActivationTime=update diagram  Latency=0  AutoFrameSizeCalculation=off
  False_3V2 : $bdroot/ThreeValuedAssistants/False_3V  SystemSampleTime=-1  VariantActivationTime=update diagram  Latency=0  AutoFrameSizeCalculation=off
  Switch3 : Switch  Criteria=u2 > Threshold
  Switch4 : Switch  Criteria=u2 > Threshold
  True_3V2 : $bdroot/ThreeValuedAssistants/True_3V  SystemSampleTime=-1  VariantActivationTime=update diagram  Latency=0  AutoFrameSizeCalculation=off
  True_3V3 : $bdroot/ThreeValuedAssistants/True_3V  SystemSampleTime=-1  VariantActivationTime=update diagram  Latency=0  AutoFrameSizeCalculation=off
  Unknown_3V1 : $bdroot/ThreeValuedAssistants/Unknown_3V  SystemSampleTime=-1  VariantActivationTime=update diagram  Latency=0  AutoFrameSizeCalculation=off
  Outport : Outport
  wires:
  Switch3/1 -> Outport/1
  False_3V1/1 -> Equal2/2
  Equal/1 -> Switch3/2
  "Input "/1 -> Equal2/1, Equal/1
  False_3V2/1 -> Switch3/1
  True_3V3/1 -> Equal/2
  Unknown_3V1/1 -> Switch4/3
  Switch4/1 -> Switch3/3
  True_3V2/1 -> Switch4/1
  Equal2/1 -> Switch4/2

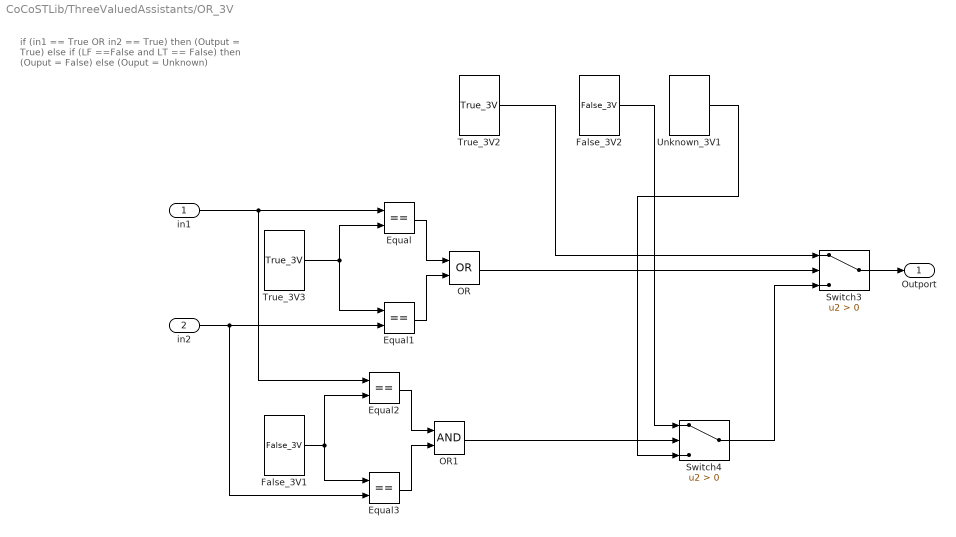
== system CoCoSTLib/ThreeValuedAssistants/OR_3V ==
  note: if (in1 == True OR in2 == True)
      | then (Output = True)
      | else if (LF ==False and LT == False)
      | then (Ouput = False)
      | else (Ouput = Unknown)
  "in1 " : Inport
  in2 : Inport  Port=2
  Equal{,1..3} (4 alike) : RelationalOperator  Operator===  OutDataTypeStr=boolean  RndMeth=Simplest
  False_3V1 : $bdroot/ThreeValuedAssistants/False_3V  SystemSampleTime=-1  VariantActivationTime=update diagram  Latency=0  AutoFrameSizeCalculation=off
  False_3V2 : $bdroot/ThreeValuedAssistants/False_3V  SystemSampleTime=-1  VariantActivationTime=update diagram  Latency=0  AutoFrameSizeCalculation=off
  OR : Logic  Operator=OR  AllPortsSameDT=off  OutDataTypeStr=boolean
  OR1 : Logic  AllPortsSameDT=off  OutDataTypeStr=boolean
  Switch3 : Switch  Criteria=u2 > Threshold
  Switch4 : Switch  Criteria=u2 > Threshold
  True_3V2 : $bdroot/ThreeValuedAssistants/True_3V  SystemSampleTime=-1  VariantActivationTime=update diagram  Latency=0  AutoFrameSizeCalculation=off
  True_3V3 : $bdroot/ThreeValuedAssistants/True_3V  SystemSampleTime=-1  VariantActivationTime=update diagram  Latency=0  AutoFrameSizeCalculation=off
  Unknown_3V1 : $bdroot/ThreeValuedAssistants/Unknown_3V  SystemSampleTime=-1  VariantActivationTime=update diagram  Latency=0  AutoFrameSizeCalculation=off
  Outport : Outport
  wires:
  True_3V3/1 -> Equal/2, Equal1/1
  Equal/1 -> OR/1
  Equal1/1 -> OR/2
  OR/1 -> Switch3/2
  Unknown_3V1/1 -> Switch4/3
  Switch3/1 -> Outport/1
  Equal2/1 -> OR1/1
  Equal3/1 -> OR1/2
  OR1/1 -> Switch4/2
  "in1 "/1 -> Equal2/1, Equal/1
  False_3V1/1 -> Equal2/2, Equal3/1
  in2/1 -> Equal1/2, Equal3/2
  False_3V2/1 -> Switch4/1
  Switch4/1 -> Switch3/3
  True_3V2/1 -> Switch3/1

== system CoCoSTLib/ThreeValuedAssistants/True_3V ==
  Constant : Constant
  Out1 : Outport
  wires:
  Constant/1 -> Out1/1

== system CoCoSTLib/ThreeValuedAssistants/Unknown_3V ==
  Constant2 : Constant  Value=-1
  Out1 : Outport
  wires:
  Constant2/1 -> Out1/1

== system CoCoSTLib/Additional/AndStl_LF/DetectDecrease ==
  note: U(k)
  note: Edge
  U : Inport
  FixPt Relational Operator : RelationalOperator  Operator=<  OutDataTypeStr=boolean  ZeroCross=off  RndMeth=Nearest
  Memory : Memory
  Y : Outport  InitialOutput=0
  wires:
  Memory/1 -> FixPt Relational Operator/2  "U(k-1)"
  FixPt Relational Operator/1 -> Y/1
  U/1 -> Memory/1, FixPt Relational Operator/1

== system CoCoSTLib/Additional/AndStl_LT/DetectIncrease ==
  note: U(k)
  note: Edge
  U : Inport
  FixPt Relational Operator : RelationalOperator  Operator=>  OutDataTypeStr=boolean  ZeroCross=off  RndMeth=Nearest
  Memory : Memory
  Y : Outport  InitialOutput=0
  wires:
  Memory/1 -> FixPt Relational Operator/2  "U(k-1)"
  FixPt Relational Operator/1 -> Y/1
  U/1 -> Memory/1, FixPt Relational Operator/1

== system CoCoSTLib/Detectors/Overshoot/Step  ==
  signal : Inport
  r : Inport  Port=2
  CMP : RelationalOperator  Operator=>  OutDataTypeStr=boolean  RndMeth=Simplest
  MEM : Memory
  SUB : Sum  Inputs=+-
  OUT : Outport
  wires:
  MEM/1 -> SUB/2
  CMP/1 -> OUT/1
  signal/1 -> MEM/1, SUB/1
  SUB/1 -> CMP/1
  r/1 -> CMP/2

== system CoCoSTLib/Detectors/Ring_once/Fall ==
  signal : Inport
  a : Inport  Port=2
  CMP : RelationalOperator  Operator=>  OutDataTypeStr=boolean  RndMeth=Simplest
  Subtract : Sum  Inputs=+-
  Transport Delay : TransportDelay  DelayTime=d
  OUT : Outport
  wires:
  CMP/1 -> OUT/1
  Transport Delay/1 -> Subtract/1  "s(t-d)"
  Subtract/1 -> CMP/1
  a/1 -> CMP/2
  signal/1 -> Subtract/2, Transport Delay/1

== system CoCoSTLib/Detectors/Ring_once/Rise ==
  signal : Inport
  "a " : Inport  Port=2
  CMP1 : RelationalOperator  Operator=>  OutDataTypeStr=boolean  RndMeth=Simplest
  Subtract1 : Sum  Inputs=-+
  Transport Delay1 : TransportDelay  DelayTime=d
  OUT : Outport
  wires:
  "a "/1 -> CMP1/2
  signal/1 -> Subtract1/2, Transport Delay1/1
  Transport Delay1/1 -> Subtract1/1  "s(t-d)"
  Subtract1/1 -> CMP1/1
  CMP1/1 -> OUT/1

== system CoCoSTLib/Detectors/RiseTime/Step  ==
  signal : Inport
  r : Inport  Port=2
  CMP : RelationalOperator  Operator=>  OutDataTypeStr=boolean  RndMeth=Simplest
  MEM : Memory
  SUB : Sum  Inputs=+-
  OUT : Outport
  wires:
  MEM/1 -> SUB/2
  CMP/1 -> OUT/1
  signal/1 -> MEM/1, SUB/1
  SUB/1 -> CMP/1
  r/1 -> CMP/2

== system CoCoSTLib/Detectors/SettlingTime/Step  ==
  signal : Inport
  r : Inport  Port=2
  CMP : RelationalOperator  Operator=>  OutDataTypeStr=boolean  RndMeth=Simplest
  MEM : Memory
  SUB : Sum  Inputs=+-
  OUT : Outport
  wires:
  MEM/1 -> SUB/2
  CMP/1 -> OUT/1
  signal/1 -> MEM/1, SUB/1
  SUB/1 -> CMP/1
  r/1 -> CMP/2

== system CoCoSTLib/Operators/Operators_3V/Always_3V ==
  "T_start " : Inport
  "T_end " : Inport  Port=2
  P : Inport  Port=3
  Always LF : $bdroot/Operators/Operators_LF/Always_LF  SystemSampleTime=-1  VariantActivationTime=update diagram  Latency=0  AutoFrameSizeCalculation=off
  "Always LT " : $bdroot/Operators/Operators_LT/Always_LT   SystemSampleTime=-1  VariantActivationTime=update diagram  Latency=0  AutoFrameSizeCalculation=off
  "Interpreter " : $bdroot/ThreeValuedAssistants/Interpreter   SystemSampleTime=-1  VariantActivationTime=update diagram  Latency=0  AutoFrameSizeCalculation=off
  3V : Outport
  wires:
  "T_end "/1 -> "Always LT "/2, Always LF/2
  Always LF/1 -> "Interpreter "/1
  "Interpreter "/1 -> 3V/1
  "T_start "/1 -> Always LF/1, "Always LT "/1
  P/1 -> Always LF/3, "Always LT "/3
  "Always LT "/1 -> "Interpreter "/2

== system CoCoSTLib/Operators/Operators_3V/Eventually_3V ==
  "T_start " : Inport
  "T_end " : Inport  Port=2
  P : Inport  Port=3
  Eventually LF : $bdroot/Operators/Operators_LF/Eventually_LF  SystemSampleTime=-1  VariantActivationTime=update diagram  Latency=0  AutoFrameSizeCalculation=off
  "Eventually LT " : $bdroot/Operators/Operators_LT/Eventually_LT   SystemSampleTime=-1  VariantActivationTime=update diagram  Latency=0  AutoFrameSizeCalculation=off
  "Interpreter " : $bdroot/ThreeValuedAssistants/Interpreter   SystemSampleTime=-1  VariantActivationTime=update diagram  Latency=0  AutoFrameSizeCalculation=off
  3V : Outport
  wires:
  Eventually LF/1 -> "Interpreter "/1
  "Eventually LT "/1 -> "Interpreter "/2
  P/1 -> "Eventually LT "/3, Eventually LF/3
  "T_end "/1 -> "Eventually LT "/2, Eventually LF/2
  "Interpreter "/1 -> 3V/1
  "T_start "/1 -> "Eventually LT "/1, Eventually LF/1

== system CoCoSTLib/Operators/Operators_3V/Until_3V ==
  "T_start " : Inport
  "T_end " : Inport  Port=2
  P : Inport  Port=3
  "Q " : Inport  Port=4
  "Interpreter " : $bdroot/ThreeValuedAssistants/Interpreter   SystemSampleTime=-1  VariantActivationTime=update diagram  Latency=0  AutoFrameSizeCalculation=off
  Until LF : $bdroot/Operators/Operators_LF/Until_LF  SystemSampleTime=-1  VariantActivationTime=update diagram  Latency=0  AutoFrameSizeCalculation=off
  Until LT : $bdroot/Operators/Operators_LT/Until_LT  SystemSampleTime=-1  VariantActivationTime=update diagram  Latency=0  AutoFrameSizeCalculation=off
  3V : Outport
  wires:
  "T_end "/1 -> Until LF/2, Until LT/2
  "T_start "/1 -> Until LT/1, Until LF/1
  "Q "/1 -> Until LF/4, Until LT/4
  P/1 -> Until LF/3, Until LT/3
  "Interpreter "/1 -> 3V/1
  Until LT/1 -> "Interpreter "/2
  Until LF/1 -> "Interpreter "/1

== system CoCoSTLib/Operators/Operators_LF/Always_LF ==
  note: DESIGN
      | If t in timewindow, output = signal AND timewindow
      | Otherwise , output = 1
  T_Start : Inport
  T_End : Inport  Port=2
  P : Inport  Port=3
  AND : Logic  AllPortsSameDT=off  OutDataTypeStr=boolean
  AND1 : Logic  AllPortsSameDT=off  OutDataTypeStr=boolean
  CLOCK : Clock
  Constant : Constant
  Memory_init1 : Memory  InitialCondition=1
  OR : Logic  AllPortsSameDT=off  OutDataTypeStr=boolean
  REL1 : RelationalOperator  Operator=<=  OutDataTypeStr=boolean  RndMeth=Simplest
  REL2 : RelationalOperator  Operator=<=  OutDataTypeStr=boolean  RndMeth=Simplest
  Switch : Switch  Criteria=u2 > Threshold
  VALID : Outport
  wires:
  AND1/1 -> Switch/1
  CLOCK/1 -> REL2/1, REL1/2
  Memory_init1/1 -> OR/2
  Switch/1 -> OR/1
  T_End/1 -> REL2/2
  OR/1 -> VALID/1, Memory_init1/1
  T_Start/1 -> REL1/1
  Constant/1 -> Switch/3
  REL1/1 -> AND/1
  REL2/1 -> AND/2
  AND/1 -> AND1/2, Switch/2
  P/1 -> AND1/1

== system CoCoSTLib/Operators/Operators_LF/Always_LF_delay ==
  T_Start : Inport
  T_End : Inport  Port=2
  Delay : Inport  Port=3
  P : Inport  Port=4
  Always_LF1 : $bdroot/Operators/Operators_LF/Always_LF  SystemSampleTime=-1  VariantActivationTime=update diagram  Latency=0  AutoFrameSizeCalculation=off
  Clock : Clock
  Compare To Constant : simulink/Logic and Bit Operations/Compare To Constant  relop=>=  const=0  OutDataTypeStr=boolean
  Constant : Constant  Value=65535
  Subtract : Sum
  Subtract1 : Sum
  Subtract2 : Sum  Inputs=-+
  Switch1 : Switch  Criteria=u2 > Threshold
  Out1 : Outport
  wires:
  Subtract1/1 -> Always_LF1/2
  Always_LF1/1 -> Out1/1
  Subtract/1 -> Always_LF1/1
  Switch1/1 -> Subtract/1, Subtract1/2
  T_End/1 -> Subtract1/1
  P/1 -> Always_LF1/3
  T_Start/1 -> Subtract/2
  Clock/1 -> Subtract2/2
  Subtract2/1 -> Compare To Constant/1
  Delay/1 -> Switch1/1, Subtract2/1
  Compare To Constant/1 -> Switch1/2
  Constant/1 -> Switch1/3

== system CoCoSTLib/Operators/Operators_LF/Always_LF_param ==
  note: DESIGN
      | If t in timewindow, output = signal AND timewindow
      | Otherwise , output = 1
  P : Inport
  AND : Logic  AllPortsSameDT=off  OutDataTypeStr=boolean
  AND1 : Logic  AllPortsSameDT=off  OutDataTypeStr=boolean
  CLOCK : Clock
  Constant : Constant
  Memory_init1 : Memory  InitialCondition=1
  OR : Logic  AllPortsSameDT=off  OutDataTypeStr=boolean
  REL1 : RelationalOperator  Operator=<=  OutDataTypeStr=boolean  RndMeth=Simplest
  REL2 : RelationalOperator  Operator=<=  OutDataTypeStr=boolean  RndMeth=Simplest
  Switch : Switch  Criteria=u2 > Threshold
  T_End : Constant  Value=T_End
  T_Start : Constant  Value=T_Start
  VALID : Outport
  wires:
  Memory_init1/1 -> OR/2
  Switch/1 -> OR/1
  REL2/1 -> AND/2
  CLOCK/1 -> REL2/1, REL1/2
  T_Start/1 -> REL1/1
  AND1/1 -> Switch/1
  REL1/1 -> AND/1
  AND/1 -> AND1/2, Switch/2
  P/1 -> AND1/1
  T_End/1 -> REL2/2
  OR/1 -> VALID/1, Memory_init1/1
  Constant/1 -> Switch/3

== system CoCoSTLib/Operators/Operators_LF/Eventually_LF ==
  note: DESIGN
      | t < t_end, output = 1
      | t >= t_end, output = accumulated_signal AND timewindow
  T_Start : Inport
  T_End : Inport  Port=2
  P : Inport  Port=3
  AND1 : Logic  Inputs=3  AllPortsSameDT=off  OutDataTypeStr=boolean
  CLOCK : Clock
  Constant1 : Constant
  "Memory_init0 " : Memory
  Memory_init1 : Memory  InitialCondition=1
  OR : Logic  AllPortsSameDT=off  OutDataTypeStr=boolean
  OR1 : Logic  Operator=OR  AllPortsSameDT=off  OutDataTypeStr=boolean
  REL1 : RelationalOperator  Operator=<=  OutDataTypeStr=boolean  RndMeth=Simplest
  REL2 : RelationalOperator  Operator=<=  OutDataTypeStr=boolean  RndMeth=Simplest
  REL3 : RelationalOperator  Operator=>  OutDataTypeStr=boolean  RndMeth=Simplest
  Switch1 : Switch  Criteria=u2 > Threshold
  VALID : Outport
  wires:
  T_End/1 -> REL3/1, REL2/2
  AND1/1 -> OR1/1
  REL1/1 -> AND1/1
  P/1 -> AND1/3
  CLOCK/1 -> REL3/2, REL1/2, REL2/1
  T_Start/1 -> REL1/1
  "Memory_init0 "/1 -> OR1/2
  OR1/1 -> "Memory_init0 "/1, Switch1/3
  Constant1/1 -> Switch1/1
  REL2/1 -> AND1/2
  REL3/1 -> Switch1/2
  Memory_init1/1 -> OR/2
  OR/1 -> VALID/1, Memory_init1/1
  Switch1/1 -> OR/1

== system CoCoSTLib/Operators/Operators_LF/Eventually_LF_param ==
  note: DESIGN
      | t < t_end, output = 1
      | t >= t_end, output = accumulated_signal AND timewindow
  P : Inport
  AND1 : Logic  Inputs=3  AllPortsSameDT=off  OutDataTypeStr=boolean
  CLOCK : Clock
  Constant1 : Constant
  "Memory_init0 " : Memory
  Memory_init1 : Memory  InitialCondition=1
  OR : Logic  AllPortsSameDT=off  OutDataTypeStr=boolean
  OR1 : Logic  Operator=OR  AllPortsSameDT=off  OutDataTypeStr=boolean
  REL1 : RelationalOperator  Operator=<=  OutDataTypeStr=boolean  RndMeth=Simplest
  REL2 : RelationalOperator  Operator=<=  OutDataTypeStr=boolean  RndMeth=Simplest
  REL3 : RelationalOperator  Operator=>  OutDataTypeStr=boolean  RndMeth=Simplest
  Switch1 : Switch  Criteria=u2 > Threshold
  T_End : Constant  Value=T_End
  T_Start : Constant  Value=T_Start
  VALID : Outport
  wires:
  T_End/1 -> REL3/1, REL2/2
  AND1/1 -> OR1/1
  REL1/1 -> AND1/1
  P/1 -> AND1/3
  CLOCK/1 -> REL3/2, REL1/2, REL2/1
  T_Start/1 -> REL1/1
  "Memory_init0 "/1 -> OR1/2
  OR1/1 -> "Memory_init0 "/1, Switch1/3
  Constant1/1 -> Switch1/1
  REL2/1 -> AND1/2
  REL3/1 -> Switch1/2
  Memory_init1/1 -> OR/2
  OR/1 -> VALID/1, Memory_init1/1
  Switch1/1 -> OR/1

== system CoCoSTLib/Operators/Operators_LF/Eventually_LFbis ==
  note: DESIGN
      | t < t_end, output = 1
      | t >= t_end, output = accumulated_signal AND timewindow
  T_Start : Inport
  T_End : Inport  Port=2
  P : Inport  Port=3
  AND2 : Logic  AllPortsSameDT=off  OutDataTypeStr=boolean
  Always LF : $bdroot/Operators_LF/Always_LF  SystemSampleTime=-1  Latency=0  AutoFrameSizeCalculation=off
  CLOCK1 : Clock
  Memory_init1 : Memory  InitialCondition=1
  NOT : Logic  Operator=NOT  IconShape=distinctive  AllPortsSameDT=off  OutDataTypeStr=boolean
  NOT1 : Logic  Operator=NOT  IconShape=distinctive  AllPortsSameDT=off  OutDataTypeStr=boolean
  OR : Logic  AllPortsSameDT=off  OutDataTypeStr=boolean
  REL4 : RelationalOperator  Operator=<=  OutDataTypeStr=boolean  RndMeth=Simplest
  VALID : Outport
  wires:
  T_Start/1 -> Always LF/1
  T_End/1 -> Always LF/2, REL4/1
  P/1 -> NOT/1
  NOT/1 -> Always LF/3
  CLOCK1/1 -> REL4/2
  Always LF/1 -> AND2/1
  REL4/1 -> AND2/2
  AND2/1 -> NOT1/1
  Memory_init1/1 -> OR/2
  NOT1/1 -> OR/1
  OR/1 -> VALID/1, Memory_init1/1

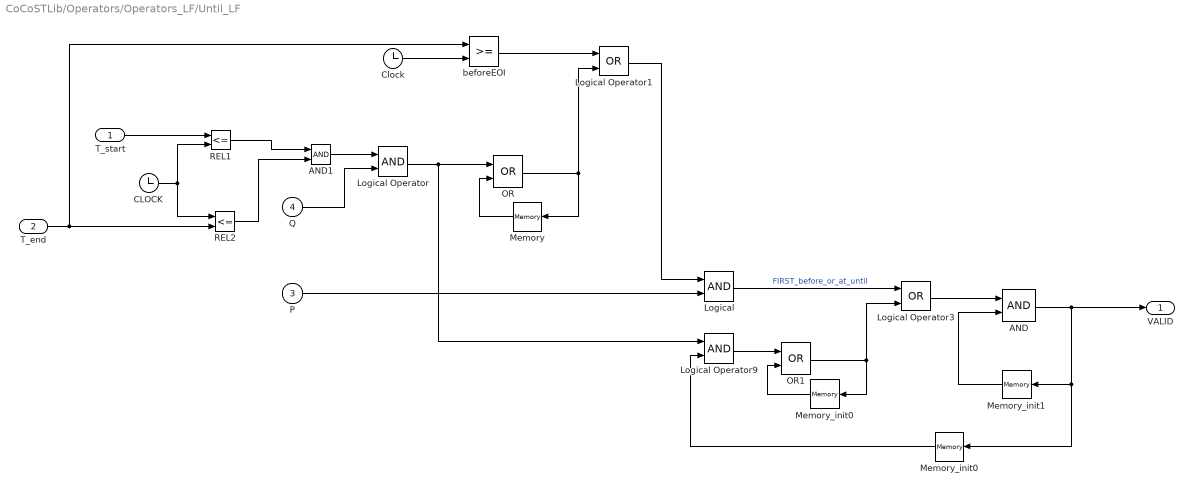
== system CoCoSTLib/Operators/Operators_LF/Until_LF ==
  "T_start " : Inport
  T_end : Inport  Port=2
  P : Inport  Port=3
  Q : Inport  Port=4
  AND : Logic  AllPortsSameDT=off  OutDataTypeStr=boolean
  AND1 : Logic  AllPortsSameDT=off  OutDataTypeStr=boolean
  CLOCK : Clock
  Clock : Clock
  "Logical " : Logic  AllPortsSameDT=off  OutDataTypeStr=boolean
  Logical Operator : Logic  AllPortsSameDT=off  OutDataTypeStr=boolean
  Logical Operator1 : Logic  Operator=OR  AllPortsSameDT=off  OutDataTypeStr=boolean
  Logical Operator3 : Logic  Operator=OR  AllPortsSameDT=off  OutDataTypeStr=boolean
  Logical Operator9 : Logic  AllPortsSameDT=off  OutDataTypeStr=boolean
  Memory : Memory
  Memory_init0 : Memory
  "Memory_init0 " : Memory
  Memory_init1 : Memory  InitialCondition=1
  OR : Logic  Operator=OR  AllPortsSameDT=off  OutDataTypeStr=boolean
  OR1 : Logic  Operator=OR  AllPortsSameDT=off  OutDataTypeStr=boolean
  REL1 : RelationalOperator  Operator=<=  OutDataTypeStr=boolean  RndMeth=Simplest
  REL2 : RelationalOperator  Operator=<=  OutDataTypeStr=boolean  RndMeth=Simplest
  beforeEOI : RelationalOperator  OutDataTypeStr=boolean  RndMeth=Nearest
  VALID : Outport
  wires:
  Memory_init0/1 -> OR1/2
  Logical Operator1/1 -> "Logical "/1
  beforeEOI/1 -> Logical Operator1/1
  REL2/1 -> AND1/2
  P/1 -> "Logical "/2
  AND1/1 -> Logical Operator/1
  Logical Operator3/1 -> AND/1
  REL1/1 -> AND1/1
  OR/1 -> Memory/1, Logical Operator1/2
  "Logical "/1 -> Logical Operator3/1  "FIRST_before_or_at_until"
  "T_start "/1 -> REL1/1
  Logical Operator9/1 -> OR1/1
  AND/1 -> VALID/1, "Memory_init0 "/1, Memory_init1/1
  Logical Operator/1 -> OR/1, Logical Operator9/1
  Memory/1 -> OR/2
  CLOCK/1 -> REL2/1, REL1/2
  Q/1 -> Logical Operator/2
  "Memory_init0 "/1 -> Logical Operator9/2
  T_end/1 -> beforeEOI/1, REL2/2
  OR1/1 -> Memory_init0/1, Logical Operator3/2
  Memory_init1/1 -> AND/2
  Clock/1 -> beforeEOI/2

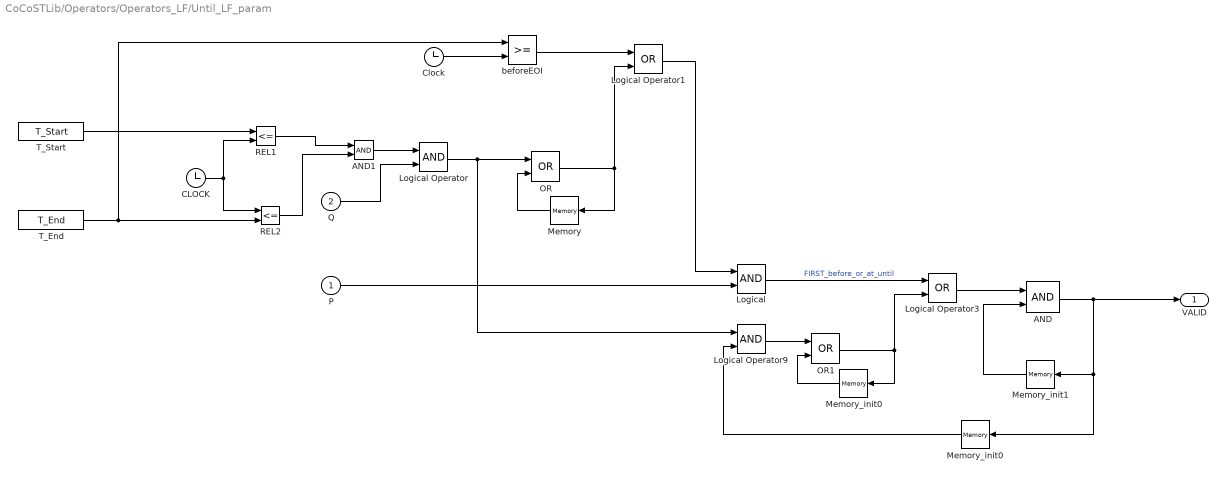
== system CoCoSTLib/Operators/Operators_LF/Until_LF_param ==
  P : Inport
  Q : Inport  Port=2
  AND : Logic  AllPortsSameDT=off  OutDataTypeStr=boolean
  AND1 : Logic  AllPortsSameDT=off  OutDataTypeStr=boolean
  CLOCK : Clock
  Clock : Clock
  "Logical " : Logic  AllPortsSameDT=off  OutDataTypeStr=boolean
  Logical Operator : Logic  AllPortsSameDT=off  OutDataTypeStr=boolean
  Logical Operator1 : Logic  Operator=OR  AllPortsSameDT=off  OutDataTypeStr=boolean
  Logical Operator3 : Logic  Operator=OR  AllPortsSameDT=off  OutDataTypeStr=boolean
  Logical Operator9 : Logic  AllPortsSameDT=off  OutDataTypeStr=boolean
  Memory : Memory
  Memory_init0 : Memory
  "Memory_init0 " : Memory
  Memory_init1 : Memory  InitialCondition=1
  OR : Logic  Operator=OR  AllPortsSameDT=off  OutDataTypeStr=boolean
  OR1 : Logic  Operator=OR  AllPortsSameDT=off  OutDataTypeStr=boolean
  REL1 : RelationalOperator  Operator=<=  OutDataTypeStr=boolean  RndMeth=Simplest
  REL2 : RelationalOperator  Operator=<=  OutDataTypeStr=boolean  RndMeth=Simplest
  T_End : Constant  Value=T_End
  T_Start : Constant  Value=T_Start
  beforeEOI : RelationalOperator  OutDataTypeStr=boolean  RndMeth=Nearest
  VALID : Outport
  wires:
  Memory_init1/1 -> AND/2
  REL2/1 -> AND1/2
  AND1/1 -> Logical Operator/1
  Memory/1 -> OR/2
  P/1 -> "Logical "/2
  "Logical "/1 -> Logical Operator3/1  "FIRST_before_or_at_until"
  Q/1 -> Logical Operator/2
  Logical Operator1/1 -> "Logical "/1
  Clock/1 -> beforeEOI/2
  AND/1 -> VALID/1, "Memory_init0 "/1, Memory_init1/1
  CLOCK/1 -> REL2/1, REL1/2
  "Memory_init0 "/1 -> Logical Operator9/2
  Logical Operator9/1 -> OR1/1
  REL1/1 -> AND1/1
  OR/1 -> Memory/1, Logical Operator1/2
  beforeEOI/1 -> Logical Operator1/1
  Memory_init0/1 -> OR1/2
  Logical Operator3/1 -> AND/1
  OR1/1 -> Memory_init0/1, Logical Operator3/2
  T_End/1 -> beforeEOI/1, REL2/2
  T_Start/1 -> REL1/1
  Logical Operator/1 -> OR/1, Logical Operator9/1

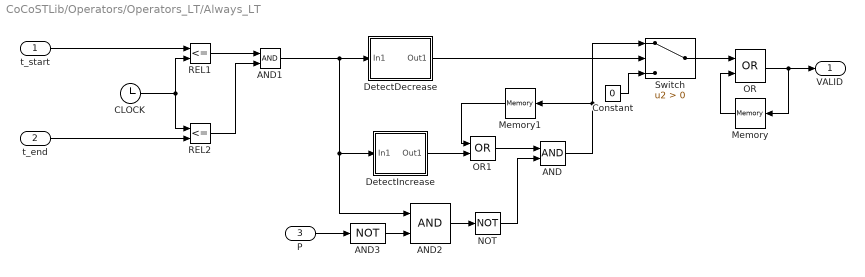
== system CoCoSTLib/Operators/Operators_LT/Always_LT  ==
  t_start : Inport
  t_end : Inport  Port=2
  P : Inport  Port=3
  AND : Logic  AllPortsSameDT=off  OutDataTypeStr=boolean
  AND1 : Logic  AllPortsSameDT=off  OutDataTypeStr=boolean
  AND2 : Logic  AllPortsSameDT=off  OutDataTypeStr=boolean
  AND3 : Logic  Operator=NOT  AllPortsSameDT=off  OutDataTypeStr=boolean
  CLOCK : Clock
  Constant : Constant  Value=0  OutDataTypeStr=boolean
  "DetectDecrease " : Subsystem
  DetectIncrease : Subsystem
  Memory : Memory
  Memory1 : Memory
  NOT : Logic  Operator=NOT  AllPortsSameDT=off  OutDataTypeStr=boolean
  OR : Logic  Operator=OR  AllPortsSameDT=off  OutDataTypeStr=boolean
  OR1 : Logic  Operator=OR  AllPortsSameDT=off  OutDataTypeStr=boolean
  REL1 : RelationalOperator  Operator=<=  OutDataTypeStr=boolean  RndMeth=Simplest
  REL2 : RelationalOperator  Operator=<=  OutDataTypeStr=boolean  RndMeth=Simplest
  Switch : Switch  Criteria=u2 > Threshold
  VALID : Outport
  wires:
  OR/1 -> Memory/1, VALID/1
  NOT/1 -> AND/2
  AND3/1 -> AND2/2
  Memory/1 -> OR/2
  AND/1 -> Memory1/1, Switch/1
  OR1/1 -> AND/1
  P/1 -> AND3/1
  Memory1/1 -> OR1/1
  AND2/1 -> NOT/1
  Switch/1 -> OR/1
  Constant/1 -> Switch/3
  t_end/1 -> REL2/2
  CLOCK/1 -> REL1/2, REL2/1
  REL2/1 -> AND1/2
  REL1/1 -> AND1/1
  t_start/1 -> REL1/1
  "DetectDecrease "/1(Out1) -> Switch/2
  AND1/1 -> AND2/1, DetectIncrease/1(In1), "DetectDecrease "/1(In1)
  DetectIncrease/1(Out1) -> OR1/2

== system CoCoSTLib/Operators/Operators_LT/Always_LT_timewindow ==
  Timewindow : Inport
  P : Inport  Port=2
  AND : Logic  AllPortsSameDT=off  OutDataTypeStr=boolean
  AND2 : Logic  AllPortsSameDT=off  OutDataTypeStr=boolean
  AND3 : Logic  Operator=NOT  AllPortsSameDT=off  OutDataTypeStr=boolean
  Constant : Constant  Value=0  OutDataTypeStr=boolean
  DetectDecrease : Subsystem
  DetectIncrease : Subsystem
  Memory : Memory
  Memory1 : Memory
  NOT : Logic  Operator=NOT  AllPortsSameDT=off  OutDataTypeStr=boolean
  OR : Logic  Operator=OR  AllPortsSameDT=off  OutDataTypeStr=boolean
  OR1 : Logic  Operator=OR  AllPortsSameDT=off  OutDataTypeStr=boolean
  Switch : Switch  Criteria=u2 > Threshold
  VALID : Outport
  wires:
  AND2/1 -> NOT/1
  DetectIncrease/1(Out1) -> OR1/2
  DetectDecrease/1(Out1) -> Switch/2
  AND/1 -> Memory1/1, Switch/1
  AND3/1 -> AND2/2
  Timewindow/1 -> AND2/1, DetectIncrease/1(In1), DetectDecrease/1(In1)
  P/1 -> AND3/1
  Constant/1 -> Switch/3
  Switch/1 -> OR/1
  OR/1 -> Memory/1, VALID/1
  Memory/1 -> OR/2
  Memory1/1 -> OR1/1
  OR1/1 -> AND/1
  NOT/1 -> AND/2

== system CoCoSTLib/Operators/Operators_LT/Always_LTbis ==
  T_Start : Inport
  T_End : Inport  Port=2
  P : Inport  Port=3
  AND2 : Logic  Inputs=3  AllPortsSameDT=off  OutDataTypeStr=boolean
  CLOCK : Clock
  Memory : Memory
  NOT : Logic  Operator=NOT  IconShape=distinctive  AllPortsSameDT=off  OutDataTypeStr=boolean
  NOT1 : Logic  Operator=NOT  IconShape=distinctive  AllPortsSameDT=off  OutDataTypeStr=boolean
  OR : Logic  Operator=OR  AllPortsSameDT=off  OutDataTypeStr=boolean
  REL1 : RelationalOperator  Operator=<=  OutDataTypeStr=boolean  RndMeth=Simplest
  REL2 : RelationalOperator  Operator=<=  OutDataTypeStr=boolean  RndMeth=Simplest
  VALID : Outport
  wires:
  AND2/1 -> NOT/1
  P/1 -> NOT1/1
  REL1/1 -> AND2/2
  REL2/1 -> AND2/3
  T_Start/1 -> REL1/1
  T_End/1 -> REL2/2
  CLOCK/1 -> REL2/1, REL1/2
  Memory/1 -> OR/2
  OR/1 -> VALID/1, Memory/1
  NOT1/1 -> AND2/1
  NOT/1 -> OR/1

== system CoCoSTLib/Operators/Operators_LT/Eventually_LT  ==
  T_Start : Inport
  T_End : Inport  Port=2
  P : Inport  Port=3
  AND2 : Logic  Inputs=3  AllPortsSameDT=off  OutDataTypeStr=boolean
  CLOCK : Clock
  Memory : Memory
  OR : Logic  Operator=OR  AllPortsSameDT=off  OutDataTypeStr=boolean
  REL1 : RelationalOperator  Operator=<=  OutDataTypeStr=boolean  RndMeth=Simplest
  REL2 : RelationalOperator  Operator=<=  OutDataTypeStr=boolean  RndMeth=Simplest
  VALID : Outport
  wires:
  REL1/1 -> AND2/2
  T_Start/1 -> REL1/1
  P/1 -> AND2/1
  REL2/1 -> AND2/3
  T_End/1 -> REL2/2
  CLOCK/1 -> REL1/2, REL2/1
  OR/1 -> Memory/1, VALID/1
  AND2/1 -> OR/1
  Memory/1 -> OR/2

== system CoCoSTLib/Operators/Operators_LT/Eventually_LT bis ==
  T_Start : Inport
  T_End : Inport  Port=2
  P : Inport  Port=3
  AND2 : Logic  Inputs=3  AllPortsSameDT=off  OutDataTypeStr=boolean
  CLOCK : Clock
  Memory : Memory
  OR : Logic  Operator=OR  AllPortsSameDT=off  OutDataTypeStr=boolean
  REL1 : RelationalOperator  Operator=<=  OutDataTypeStr=boolean  RndMeth=Simplest
  REL2 : RelationalOperator  Operator=<=  OutDataTypeStr=boolean  RndMeth=Simplest
  VALID : Outport
  wires:
  Memory/1 -> OR/2
  AND2/1 -> OR/1
  OR/1 -> VALID/1, Memory/1
  CLOCK/1 -> REL2/1, REL1/2
  T_End/1 -> REL2/2
  REL2/1 -> AND2/3
  P/1 -> AND2/1
  T_Start/1 -> REL1/1
  REL1/1 -> AND2/2

== system CoCoSTLib/Operators/Operators_LT/Eventually_LT_timewindow ==
  "Timewindow " : Inport
  P : Inport  Port=2
  AND2 : Logic  AllPortsSameDT=off  OutDataTypeStr=boolean
  Memory : Memory
  OR : Logic  Operator=OR  AllPortsSameDT=off  OutDataTypeStr=boolean
  VALID : Outport
  wires:
  AND2/1 -> OR/1
  OR/1 -> Memory/1, VALID/1
  "Timewindow "/1 -> AND2/2
  P/1 -> AND2/1
  Memory/1 -> OR/2
